simulink subsystem "Custom"  (R2025a)
settings: Solver=VariableStepAuto  StartTime=0.0  StopTime=10.0  RelTol=1e-3
libraries: px4Utilslib x1
settings Model: Creator=gurt1  LastModifiedBy=gurt1

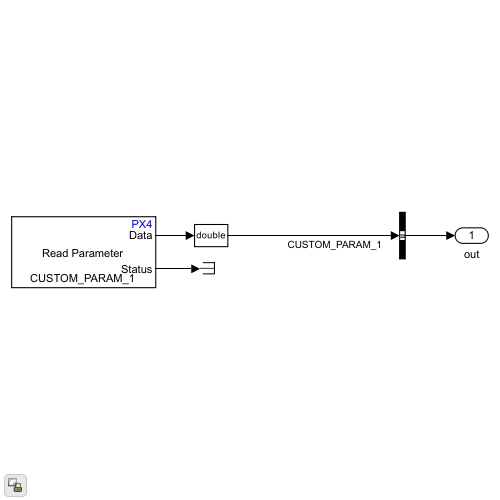
[thumbnail: Simulink's stored preview of the top-level diagram]
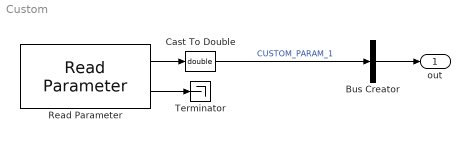
== system Custom ==
  Bus Creator : BusCreator  Inputs=1
  Cast To Double : DataTypeConversion  OutDataTypeStr=double  SaturateOnIntegerOverflow=off  RndMeth=Floor
  Read Parameter : px4Utilslib/Read Parameter  ParameterName=CUSTOM_PARAM_1  DataType=FLOAT  SampleTime=-1
  Terminator : Terminator
  out : Outport
  wires:
  Read Parameter/2 -> Terminator/1
  Read Parameter/1 -> Cast To Double/1
  Cast To Double/1 -> Bus Creator/1  "CUSTOM_PARAM_1"
  Bus Creator/1 -> out/1
